simulink model "boat_model_and_controller_inertial"  (R2021a)
settings: Solver=VariableStepAuto  StartTime=0.0  StopTime=20  FixedStep=0.01  RelTol=1e-3
undefined symbols (not defined in the file): ap2, ar2, ay2, bp2, br2, by2, DiscIntNeverNeededParam, Eff, FF_L, FF_R, initial_P, initial_Q, initial_R, initial_uspeed, initial_vspeed, initial_wspeed, initial_Z, Kih, Kir, rear_alfas, T
libraries: simulink x10, dsparch4 x3, pid_lib x1
(part 1 of 2)
settings Model: Creator=Basile  LastModifiedBy=Simão Amaro
settings SolverCC: ConcurrentTasks=on  ZeroCrossAlgorithm=Adaptive  AlgebraicLoopSolver=TrustRegion  PositivePriorityOrder=on
settings DataIOCC: ExternalInput=getinputstruct(op_trim1)  InitialState=getstatestruct(op_trim1)  SaveOutput=off  DSMLogging=off  SaveTime=off  ReturnWorkspaceOutputs=off
settings OptimizationCC: BlockReduction=off  DefaultParameterBehavior=Inlined  UseDivisionForNetSlopeComputation=on  UseFloatMulNetSlope=on  OptimizeBlockIOStorage=off  BufferReuse=off  PassReuseOutputArgsThreshold=0  EfficientFloat2IntCast=on  OptimizeBlockOrder=speed  DifferentSizesBufferReuse=on
settings DebuggingCC: InheritedTsInSrcMsg=none  ParameterTunabilityLossMsg=error  UnconnectedInputMsg=none  UnconnectedOutputMsg=none  UnconnectedLineMsg=none  UniqueDataStoreMsg=error  SFMachineParentedDataDiag=warning  ArithmeticOperatorsInVariantConditions=warning
settings HardwareCC: ProdBitPerLong=64  ProdLongLongMode=on  ProdHWDeviceType=Intel->x86-64 (Linux 64)
settings SFSimCC: SimUseLocalCustomCode=off  MATLABDynamicMemAlloc=off  CustomCodeUndefinedFunction=UseInterfaceOnly
settings RTWCC: Description=Simulink Real-Time  SystemTargetFile=slrealtime.tlc  TemplateMakefile=slrealtime_default_tmf  GenerateReport=on  RTWUseLocalCustomCode=off  Toolchain=Simulink Real-Time Toolchain  BuildConfiguration=Faster Runs  LaunchReport=on  CodeExecutionProfiling=on  TargetLang=C++
settings CodeAppCC: ForceParamTrailComments=on  OperatorAnnotations=on

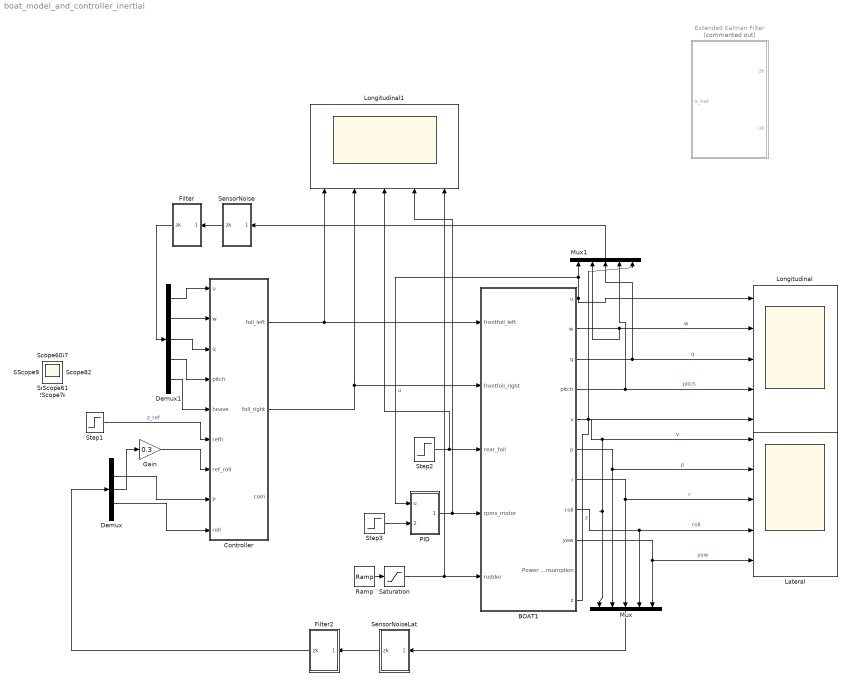
== system boat_model_and_controller_inertial ==
  BOAT1 : Subsystem
  Controller : Subsystem
  Demux : Demux  Outputs=5
  Demux1 : Demux  Outputs=5
  Extended Kalman Filter : Subsystem  Commented=on
  Filter : Subsystem
  Filter2 : Subsystem
  Gain : Gain  Gain=0.3
  Lateral : Scope  NumInputPorts=5
  Longitudinal : Scope  NumInputPorts=5
  Longitudinal1 : Scope  NumInputPorts=5
  Mux : Mux  Inputs=5
  Mux1 : Mux  Inputs=5
  PID : Subsystem
  Ramp : simulink/Sources/Ramp  slope=0  start=0  InitialOutput=15
  Saturation : Saturate  UpperLimit=15  LowerLimit=-15
  SensorNoise : Subsystem
  SensorNoiseLat : Subsystem
  Step1 : Step  Time=0  Before=initial_Z  After=-0.4  SampleTime=0
  Step2 : Step  Time=0  Before=rear_alfas  After=rear_alfas  SampleTime=0
  Step3 : Step  Time=0  Before=initial_uspeed  After=7  SampleTime=0
  Scope{,1..64} (65 alike) : Scope
  wires:
  BOAT1/2(w) -> Mux1/2, Longitudinal/2  "w"
  BOAT1/3(q) -> Mux1/3, Longitudinal/3  "q"
  BOAT1/5(v) -> Mux/1, Lateral/1  "v"
  BOAT1/6(p) -> Lateral/2, Mux/2  "p"
  BOAT1/8(roll) -> Lateral/4, Mux/4  "roll"
  BOAT1/11(z) -> Mux1/5, Longitudinal/5  "z"
  BOAT1/1(u) -> Longitudinal/1, PID/1(u), Mux1/1  "u"
  BOAT1/7(r) -> Lateral/3, Mux/3  "r"
  Demux1/2 -> Controller/2(w)
  Demux1/3 -> Controller/3(q)
  Demux1/4 -> Controller/4(pitch)
  Demux1/5 -> Controller/5(heave)
  Demux1/1 -> Controller/1(u)
  BOAT1/9(yaw) -> Mux/5, Lateral/5  "yaw"
  BOAT1/4(pitch) -> Mux1/4, Longitudinal/4  "pitch"
  Mux1/1 -> SensorNoise/1(states)
  Step1/1 -> Controller/6(refh)  "z_ref"
  Mux/1 -> SensorNoiseLat/1(states)
  Step3/1 -> PID/2(In2)
  Controller/1(foil_left) -> Longitudinal1/1, BOAT1/1(frontfoil_left)
  Controller/2(foil_right) -> Longitudinal1/2, BOAT1/2(frontfoil_right)
  Step2/1 -> Longitudinal1/3, BOAT1/3(rear_foil)
  PID/1(rpms_motor) -> BOAT1/4(rpms_motor), Longitudinal1/4
  Demux/4 -> Controller/9(roll)
  SensorNoise/1(zk) -> Filter/1(states)
  SensorNoiseLat/1(zk) -> Filter2/1(states)
  Filter/1(zk) -> Demux1/1
  Filter2/1(zk) -> Demux/1
  Gain/1 -> Controller/7(ref_roll)
  Demux/2 -> Controller/8(P)
  Demux/3 -> Gain/1
  Ramp/1 -> Saturation/1
  Saturation/1 -> BOAT1/5(rudder), Longitudinal1/5

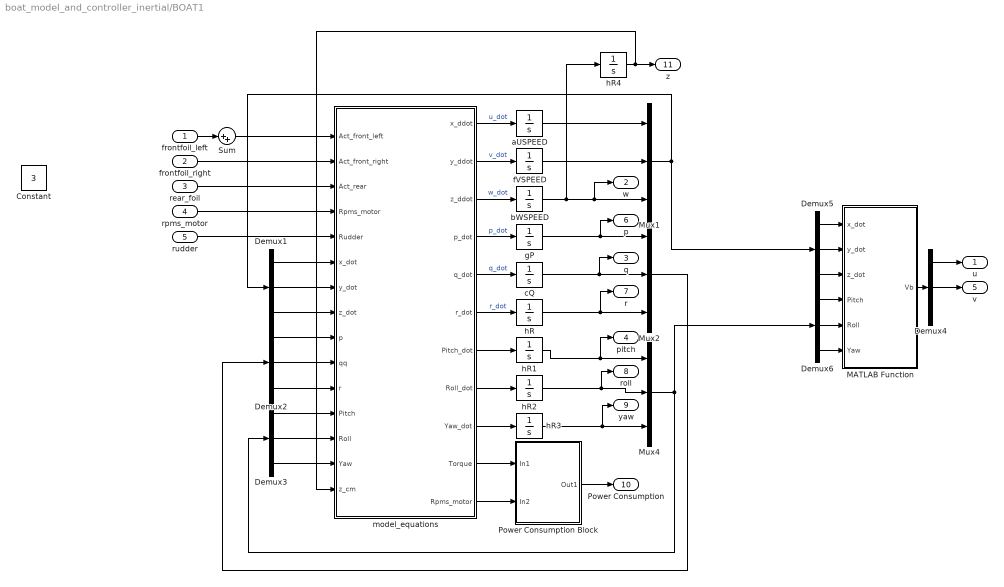
== system boat_model_and_controller_inertial/BOAT1 ==
  frontfoil_left : Inport
  frontfoil_right : Inport  Port=2
  rear_foil : Inport  Port=3
  rpms_motor : Inport  Port=4
  rudder : Inport  Port=5
  Constant : Constant  Value=3
  Demux{1..6} (6 alike) : Demux  Outputs=3
  MATLAB Function : MATLAB Function  TreatAsAtomicUnit=on
  Mux1 : Mux  Inputs=3
  Mux2 : Mux  Inputs=3
  Mux4 : Mux  Inputs=3
  Power Consumption Block : Subsystem
  Sum : Sum  Inputs=|++
  aUSPEED : Integrator  InitialCondition=initial_uspeed
  bWSPEED : Integrator  InitialCondition=initial_wspeed
  cQ : Integrator  InitialCondition=initial_Q
  fVSPEED : Integrator  InitialCondition=initial_vspeed
  gP : Integrator  InitialCondition=initial_P
  hR : Integrator  InitialCondition=initial_R
  hR1 : Integrator
  hR2 : Integrator
  hR3 : Integrator
  hR4 : Integrator  InitialCondition=initial_Z
  model_equations : MATLAB Function  TreatAsAtomicUnit=on  VariantControl=Variant1
  u : Outport  VectorParamsAs1DForOutWhenUnconnected=off
  w : Outport  Port=2  VectorParamsAs1DForOutWhenUnconnected=off
  q : Outport  Port=3  VectorParamsAs1DForOutWhenUnconnected=off
  pitch : Outport  Port=4  VectorParamsAs1DForOutWhenUnconnected=off
  v : Outport  Port=5  VectorParamsAs1DForOutWhenUnconnected=off
  p : Outport  Port=6  VectorParamsAs1DForOutWhenUnconnected=off
  r : Outport  Port=7  VectorParamsAs1DForOutWhenUnconnected=off
  roll : Outport  Port=8  VectorParamsAs1DForOutWhenUnconnected=off
  yaw : Outport  Port=9  VectorParamsAs1DForOutWhenUnconnected=off
  Power Consumption : Outport  Port=10  VectorParamsAs1DForOutWhenUnconnected=off
  z : Outport  Port=11  VectorParamsAs1DForOutWhenUnconnected=off
  wires:
  model_equations/6(r_dot) -> hR/1  "r_dot"
  Mux1/1 -> Demux5/1, Demux1/1
  model_equations/5(q_dot) -> cQ/1  "q_dot"
  rear_foil/1 -> model_equations/3(Act_rear)
  Demux3/2 -> model_equations/13(Roll)
  Demux2/2 -> model_equations/10(qq)
  Demux2/3 -> model_equations/11(r)
  model_equations/4(p_dot) -> gP/1  "p_dot"
  Demux2/1 -> model_equations/9(p)
  rpms_motor/1 -> model_equations/4("Rpms_motor ")
  Demux3/1 -> model_equations/12(Pitch)
  model_equations/2(y_ddot) -> fVSPEED/1  "v_dot"
  Demux1/2 -> model_equations/7(y_dot)
  Mux2/1 -> Demux2/1
  Demux3/3 -> model_equations/14(Yaw)
  model_equations/11(Rpms_motor) -> Power Consumption Block/2(In2)
  Power Consumption Block/1(Out1) -> Power Consumption/1
  model_equations/10(Torque) -> Power Consumption Block/1(In1)
  Demux1/1 -> model_equations/6(x_dot)
  cQ/1 -> q/1, Mux2/2
  hR/1 -> Mux2/3, r/1
  model_equations/3(z_ddot) -> bWSPEED/1  "w_dot"
  model_equations/1(x_ddot) -> aUSPEED/1  "u_dot"
  gP/1 -> p/1, Mux2/1
  model_equations/7(Pitch_dot) -> hR1/1
  model_equations/8(Roll_dot) -> hR2/1
  model_equations/9(Yaw_dot) -> hR3/1
  hR1/1 -> pitch/1, Mux4/1
  hR2/1 -> roll/1, Mux4/2
  hR3/1 -> yaw/1, Mux4/3
  Mux4/1 -> Demux6/1, Demux3/1
  rudder/1 -> model_equations/5(Rudder)
  frontfoil_right/1 -> model_equations/2(Act_front_right)
  frontfoil_left/1 -> Sum/1
  Sum/1 -> model_equations/1(Act_front_left)
  Demux1/3 -> model_equations/8(z_dot)
  fVSPEED/1 -> Mux1/2
  aUSPEED/1 -> Mux1/1
  hR4/1 -> model_equations/15(z_cm), z/1
  bWSPEED/1 -> hR4/1, w/1, Mux1/3
  MATLAB Function/1(Vb) -> Demux4/1
  Demux4/1 -> u/1
  Demux4/2 -> v/1
  Demux5/1 -> MATLAB Function/1(x_dot)
  Demux5/2 -> MATLAB Function/2(y_dot)
  Demux5/3 -> MATLAB Function/3(z_dot)
  Demux6/1 -> MATLAB Function/4(Pitch)
  Demux6/2 -> MATLAB Function/5(Roll)
  Demux6/3 -> MATLAB Function/6(Yaw)

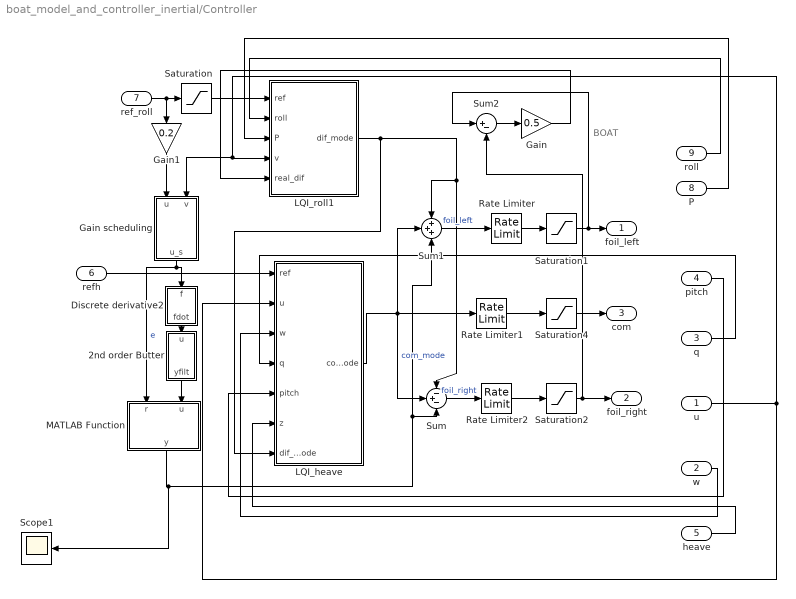
== system boat_model_and_controller_inertial/Controller ==
  note: BOAT
  u : Inport
  w : Inport  Port=2
  q : Inport  Port=3
  pitch : Inport  Port=4
  heave : Inport  Port=5
  refh : Inport  Port=6
  ref_roll : Inport  Port=7
  P : Inport  Port=8
  roll : Inport  Port=9
  2nd order Butter : Subsystem
  Discrete derivative2 : Subsystem
  Gain : Gain  Gain=0.5
  Gain scheduling : MATLAB Function  TreatAsAtomicUnit=on
  Gain1 : Gain  Gain=0.2
  LQI_heave : Subsystem  TreatAsAtomicUnit=on  SystemSampleTime=0.02
      settings: MinAlgLoopOccurrences=on
  LQI_roll1 : Subsystem  TreatAsAtomicUnit=on  SystemSampleTime=0.02
  MATLAB Function : MATLAB Function  TreatAsAtomicUnit=on
  Rate Limiter : RateLimiter  RisingSlewLimit=10  FallingSlewLimit=-10  SampleTimeMode=inherited  InitialCondition=FF_L
  Rate Limiter1 : RateLimiter  RisingSlewLimit=10  FallingSlewLimit=-10  SampleTimeMode=inherited  InitialCondition=FF_L
  Rate Limiter2 : RateLimiter  RisingSlewLimit=10  FallingSlewLimit=-10  SampleTimeMode=inherited  InitialCondition=FF_L
  Saturation : Saturate  UpperLimit=3  LowerLimit=-3
  Saturation1 : Saturate  UpperLimit=14  LowerLimit=-3
  Saturation2 : Saturate  UpperLimit=14  LowerLimit=-3
  Saturation4 : Saturate  UpperLimit=14  LowerLimit=-3
  Scope1 : Scope
  Sum : Sum  Inputs=-+-
  Sum1 : Sum  Inputs=+++
  Sum2 : Sum  Inputs=|+-
  foil_left : Outport  VectorParamsAs1DForOutWhenUnconnected=off
  foil_right : Outport  Port=2  VectorParamsAs1DForOutWhenUnconnected=off
  com : Outport  Port=3  VectorParamsAs1DForOutWhenUnconnected=off
  wires:
  LQI_heave/1(com_mode) -> Rate Limiter1/1, Sum/2, Sum1/2  "com_mode"
  roll/1 -> LQI_roll1/2(roll)
  pitch/1 -> LQI_heave/5(pitch)
  u/1 -> Gain scheduling/2(v), LQI_roll1/4(v), LQI_heave/2(u)
  w/1 -> LQI_heave/3(w)
  P/1 -> LQI_roll1/3(P)
  heave/1 -> LQI_heave/6(z)
  refh/1 -> LQI_heave/1(ref)
  Saturation1/1 -> foil_left/1, Sum2/1
  Saturation4/1 -> com/1
  ref_roll/1 -> Gain1/1, Saturation/1
  LQI_roll1/1(dif_mode) -> LQI_heave/7(dif_mode), Sum/1, Sum1/1
  q/1 -> LQI_heave/4(q)
  Rate Limiter1/1 -> Saturation4/1
  Sum/1 -> Rate Limiter2/1  "foil_right"
  Rate Limiter2/1 -> Saturation2/1
  Gain/1 -> LQI_roll1/5(real_dif)
  Sum2/1 -> Gain/1
  Sum1/1 -> Rate Limiter/1  "foil_left"
  Rate Limiter/1 -> Saturation1/1
  Saturation2/1 -> foil_right/1, Sum2/2
  Gain scheduling/1(u_s) -> Discrete derivative2/1(f), MATLAB Function/1(r)  "e"
  Discrete derivative2/1(fdot) -> 2nd order Butter/1(u)
  Gain1/1 -> Gain scheduling/1(u)
  Saturation/1 -> LQI_roll1/1(ref)
  2nd order Butter/1(yfilt) -> MATLAB Function/2(u)
  MATLAB Function/1(y) -> Scope1/1, Sum/3, Sum1/3

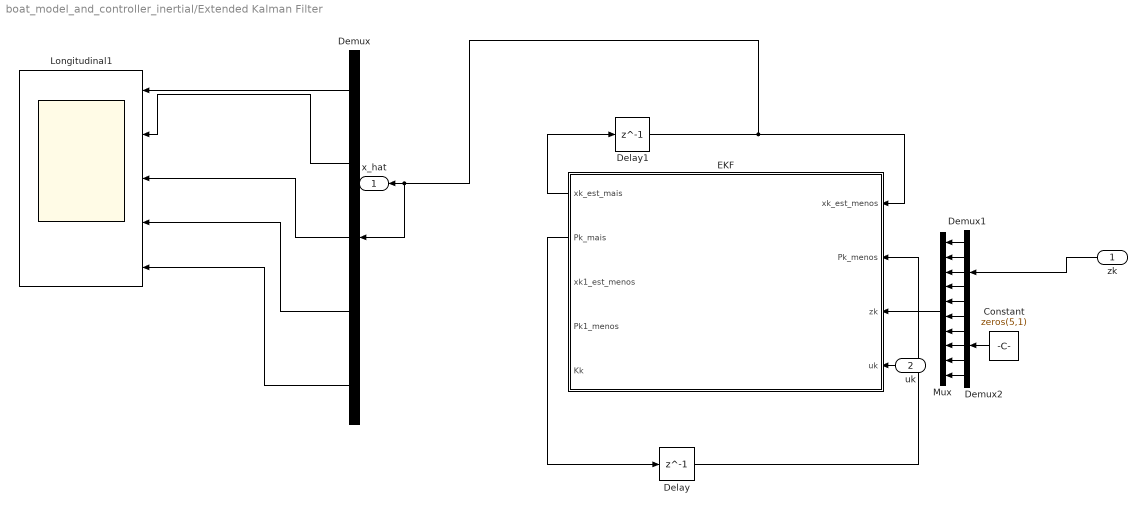
== system boat_model_and_controller_inertial/Extended Kalman Filter ==
  zk : Inport  PortDimensions=5
  uk : Inport  Port=2  PortDimensions=5
  Constant : Constant  Value=zeros(5,1)
  Delay : Delay  DelayLength=1  InitialCondition=1000*eye(37)  SampleTime=0.02
  Delay1 : Delay  DelayLength=1  InitialCondition=[initial_uspeed;0;0;0;initial_Z;0;0;0;0;0;zeros(27,1)]  SampleTime=0.02
  Demux : Demux  Outputs=5
  Demux1 : Demux  Outputs=5
  Demux2 : Demux  Outputs=5
  EKF : MATLAB Function  TreatAsAtomicUnit=on
  Longitudinal1 : Scope  NumInputPorts=5
  Mux : Mux  Inputs=10
  x_hat : Outport
  wires:
  uk/1 -> EKF/4(uk)
  Delay/1 -> EKF/2(Pk_menos)
  Demux/1 -> Longitudinal1/1
  Demux/2 -> Longitudinal1/2
  Demux/3 -> Longitudinal1/3
  Demux/4 -> Longitudinal1/4
  Demux/5 -> Longitudinal1/5
  Delay1/1 -> Demux/1, x_hat/1, EKF/1(xk_est_menos)
  EKF/2(Pk_mais) -> Delay/1
  EKF/1(xk_est_mais) -> Delay1/1
  zk/1 -> Demux1/1
  Mux/1 -> EKF/3(zk)
  Demux1/1 -> Mux/1
  Demux1/2 -> Mux/2
  Demux1/3 -> Mux/3
  Demux1/4 -> Mux/4
  Demux1/5 -> Mux/5
  Demux2/1 -> Mux/6
  Demux2/2 -> Mux/7
  Demux2/3 -> Mux/8
  Demux2/4 -> Mux/9
  Demux2/5 -> Mux/10
  Constant/1 -> Demux2/1

== system boat_model_and_controller_inertial/Filter ==
  states : Inport
  2nd order Butter : Subsystem
  Demux2 : Demux  Outputs=5
  Longitudinal1 : Scope  NumInputPorts=5
  Mux1 : Mux  Inputs=2
  Mux2 : Mux  Inputs=5
  zk : Outport
  wires:
  states/1 -> Demux2/1
  Mux2/1 -> zk/1
  Demux2/1 -> Mux2/1
  Demux2/2 -> Mux2/2
  Demux2/4 -> Mux2/4
  Demux2/5 -> Mux2/5
  Mux1/1 -> Longitudinal1/3
  2nd order Butter/1(yfilt) -> Mux1/1, Mux2/3
  Demux2/3 -> Mux1/2, 2nd order Butter/1(u)  "q"

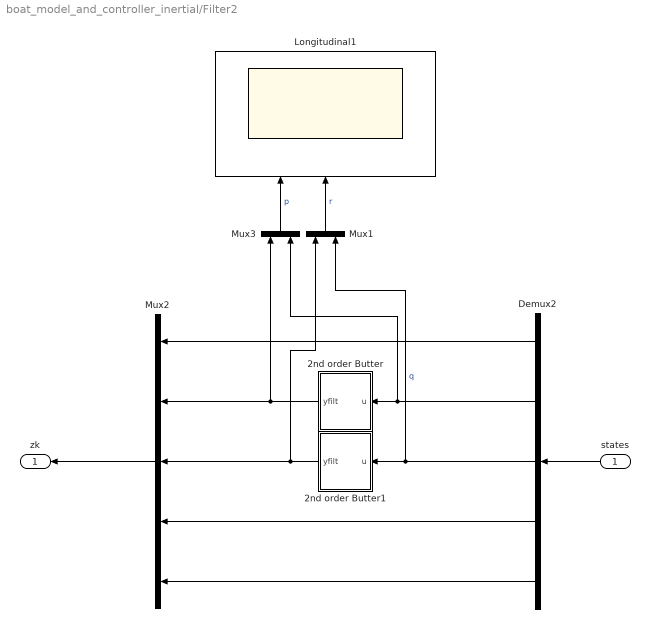
== system boat_model_and_controller_inertial/Filter2 ==
  states : Inport
  2nd order Butter : Subsystem
  2nd order Butter1 : Subsystem
  Demux2 : Demux  Outputs=5
  Longitudinal1 : Scope  NumInputPorts=5
  Mux1 : Mux  Inputs=2
  Mux2 : Mux  Inputs=5
  Mux3 : Mux  Inputs=2
  zk : Outport
  wires:
  states/1 -> Demux2/1
  Mux2/1 -> zk/1
  Demux2/1 -> Mux2/1
  Demux2/4 -> Mux2/4
  Demux2/5 -> Mux2/5
  Demux2/2 -> Mux3/2, 2nd order Butter/1(u)
  2nd order Butter/1(yfilt) -> Mux3/1, Mux2/2
  2nd order Butter1/1(yfilt) -> Mux1/1, Mux2/3
  Demux2/3 -> Mux1/2, 2nd order Butter1/1(u)  "q"
  Mux1/1 -> Longitudinal1/3  "r"
  Mux3/1 -> Longitudinal1/2  "p"

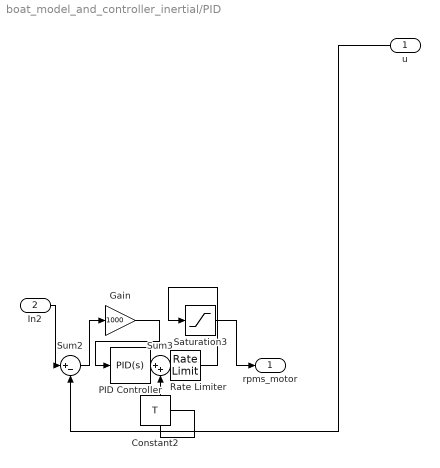
== system boat_model_and_controller_inertial/PID ==
  u : Inport
  In2 : Inport  Port=2
  Constant2 : Constant  Value=T
  Gain : Gain  Gain=1000
  PID Controller : pid_lib/PID Controller  Controller=PID  Form=Parallel  TimeDomain=Continuous-time  UseExternalTs=off  SampleTime=-1  IntegratorMethod=Forward Euler  FilterMethod=Forward Euler  ControllerParametersSource=internal  P=1  I=1  D=0.00001  UseFilter=on  N=100  TunerSelectOption=Transfer Function Based (PID Tuner App)  InitialConditionSource=internal  InitialConditionForIntegrator=0  InitialConditionForFilter=0  DifferentiatorICPrevScaledInput=0  ExternalReset=none  TrackingMode=off  Kt=1  LimitOutput=off  SatLimitsSource=internal  UpperSaturationLimit=inf  LowerSaturationLimit=-inf  LinearizeAsGain=on  AntiWindupMode=none  Kb=1  POutMin=[]  POutMax=[]  IOutMin=[]  IOutMax=[]  DOutMin=[]  DOutMax=[]  NOutMin=[]  NOutMax=[]  SumOutMin=[]  SumOutMax=[]  SaturationOutMin=[]  SaturationOutMax=[]  PParamMin=[]  PParamMax=[]  IParamMin=[]  IParamMax=[]  DParamMin=[]  DParamMax=[]  NParamMin=[]  NParamMax=[]  KbParamMin=[]  KbParamMax=[]  KtParamMin=[]  KtParamMax=[]  KbOutMin=[]  KbOutMax=[]  KtOutMin=[]  KtOutMax=[]  IntegratorOutMin=[]  IntegratorOutMax=[]  FilterOutMin=[]  FilterOutMax=[]  SumI1OutMin=[]  SumI1OutMax=[]  SumI2OutMin=[]  SumI2OutMax=[]  SumI3OutMin=[]  SumI3OutMax=[]  SumI4OutMin=[]  SumI4OutMax=[]  SumDOutMin=[]  SumDOutMax=[]  DifferentiatorOutMin=[]  DifferentiatorOutMax=[]  FilterDiffOutCoefMin=[]  FilterDiffOutCoefMax=[]  ReciprocalOutMin=[]  ReciprocalOutMax=[]  SumDenOutMin=[]  SumDenOutMax=[]  SumNumOutMin=[]  SumNumOutMax=[]  DivideOutMin=[]  DivideOutMax=[]  UdiffTsProdOutMin=[]  UdiffTsProdOutMax=[]  NTsProdOutMin=[]  NTsProdOutMax=[]  UintegralTsProdOutMin=[]  UintegralTsProdOutMax=[]  UngainTsProdOutMin=[]  UngainTsProdOutMax=[]  IntegratorContinuousStateAttributes=''  IntegratorStateMustResolveToSignalObject=off  IntegratorRTWStateStorageClass=Auto  FilterContinuousStateAttributes=''  FilterStateMustResolveToSignalObject=off  FilterRTWStateStorageClass=Auto  ParallelPVariant=InternalParameters  IdealPVariant=Disabled  IVariant=InternalParameters  DVariant=InternalParameters  IntegratorVariant=Continuous  SatVariant=Disabled  AWVariant=Passthrough  PCopyVariant=Disabled  TRVariant=Disabled  FdbkBlocksVariant=Forward  IdealPFdbkVariant=Disabled  SatFdbkVariant=Disabled  DerivativeFilterVariant=ContFilter  NVariant=InternalParameters  NCopyVariant=Disabled  FilterICVariant=InternalICsFilter  IntegratorICVariant=InternalICs  ExternalResetVariant=Disabled  TRSumVariant=Passthrough  SumFdbkVariant=Disabled  SumVariant=Sum_PID  TsampFilterVariant=InternalTs  TsampNgainVariant=Passthrough  TsampIntegralVariant=Passthrough  ExternalSaturationOutDataTypeStr=Inherit: Same as second input
  Rate Limiter : RateLimiter  RisingSlewLimit=1000  FallingSlewLimit=-1000  SampleTimeMode=inherited  InitialCondition=T
  Saturation3 : Saturate  UpperLimit=9000
  Sum2 : Sum  Inputs=|+-
  Sum3 : Sum  Inputs=|++
  rpms_motor : Outport
  wires:
  u/1 -> Sum2/2
  Sum3/1 -> Rate Limiter/1
  Gain/1 -> PID Controller/1
  Saturation3/1 -> rpms_motor/1
  PID Controller/1 -> Sum3/1
  Rate Limiter/1 -> Saturation3/1
  Sum2/1 -> Gain/1
  In2/1 -> Sum2/1
  Constant2/1 -> Sum3/2

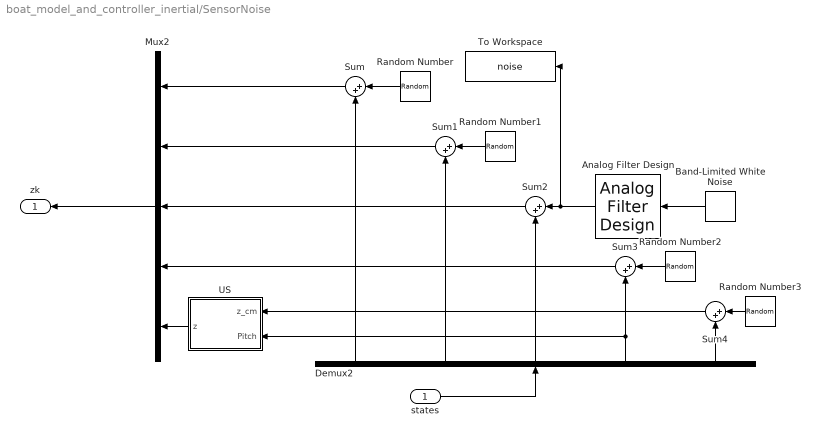
== system boat_model_and_controller_inertial/SensorNoise ==
  states : Inport
  Analog Filter Design : dsparch4/Analog Filter Design  method=Butterworth  filttype=Highpass  N=8  Wlo=3*2*pi  Whi=80  Rp=2  Rs=40
  Band-Limited White Noise : simulink/Sources/Band-Limited White Noise  Cov=[0.05]  Ts=0.02  seed=[23341]
  Demux2 : Demux  Outputs=5
  Mux2 : Mux  Inputs=5
  Random Number : RandomNumber  Variance=0.001^2  Seed=31233  SampleTime=0.02
  Random Number1 : RandomNumber  Variance=0.001^2  Seed=31232  SampleTime=0.02
  Random Number2 : RandomNumber  Variance=0.005^2  Seed=372323  SampleTime=0.02
  Random Number3 : RandomNumber  Variance=0.0005^2  Seed=312392  SampleTime=0.02
  Sum{,1..4} (5 alike) : Sum  Inputs=|++
  To Workspace : ToWorkspace  VariableName=noise  SaveFormat=Timeseries  SampleTime=0.02
  US : MATLAB Function  TreatAsAtomicUnit=on
  zk : Outport
  wires:
  Demux2/1 -> Sum/2
  Random Number2/1 -> Sum3/1
  Random Number3/1 -> Sum4/1
  Random Number/1 -> Sum/1
  Demux2/4 -> Sum3/2, US/2(Pitch)
  Demux2/3 -> Sum2/2
  Demux2/5 -> Sum4/2
  Demux2/2 -> Sum1/2
  Random Number1/1 -> Sum1/1
  states/1 -> Demux2/1
  Mux2/1 -> zk/1
  Sum/1 -> Mux2/1
  Sum1/1 -> Mux2/2
  Sum2/1 -> Mux2/3
  Sum3/1 -> Mux2/4
  US/1(z) -> Mux2/5
  Sum4/1 -> US/1(z_cm)
  Analog Filter Design/1 -> To Workspace/1, Sum2/1
  Band-Limited White Noise/1 -> Analog Filter Design/1

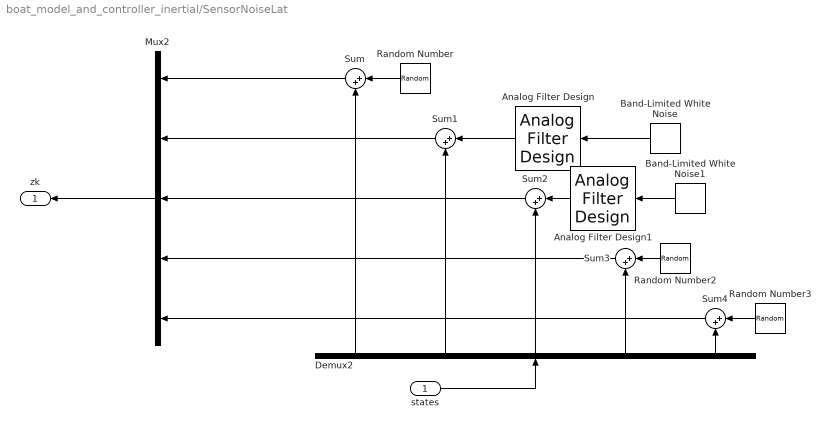
== system boat_model_and_controller_inertial/SensorNoiseLat ==
  states : Inport
  Analog Filter Design : dsparch4/Analog Filter Design  method=Butterworth  filttype=Highpass  N=8  Wlo=15*2*pi  Whi=80  Rp=2  Rs=40
  Analog Filter Design1 : dsparch4/Analog Filter Design  method=Butterworth  filttype=Highpass  N=8  Wlo=3*2*pi  Whi=80  Rp=2  Rs=40
  Band-Limited White Noise : simulink/Sources/Band-Limited White Noise  Cov=[0.0000000001]  Ts=0.02  seed=[23341]
  Band-Limited White Noise1 : simulink/Sources/Band-Limited White Noise  Cov=[0.00005]  Ts=0.02  seed=[23341]
  Demux2 : Demux  Outputs=5
  Mux2 : Mux  Inputs=5
  Random Number : RandomNumber  Variance=0.05^2  Seed=31233  SampleTime=0.02
  Random Number2 : RandomNumber  Variance=0.005^2  Seed=372323  SampleTime=0.02
  Random Number3 : RandomNumber  Variance=0.005^2  Seed=312392  SampleTime=0.02
  Sum{,1..4} (5 alike) : Sum  Inputs=|++
  zk : Outport
  wires:
  Demux2/1 -> Sum/2
  Random Number2/1 -> Sum3/1
  Random Number3/1 -> Sum4/1
  Random Number/1 -> Sum/1
  Demux2/4 -> Sum3/2
  Demux2/3 -> Sum2/2
  Demux2/5 -> Sum4/2
  Demux2/2 -> Sum1/2
  states/1 -> Demux2/1
  Mux2/1 -> zk/1
  Sum/1 -> Mux2/1
  Sum1/1 -> Mux2/2
  Sum2/1 -> Mux2/3
  Sum3/1 -> Mux2/4
  Sum4/1 -> Mux2/5
  Band-Limited White Noise/1 -> Analog Filter Design/1
  Band-Limited White Noise1/1 -> Analog Filter Design1/1
  Analog Filter Design1/1 -> Sum2/1
  Analog Filter Design/1 -> Sum1/1

== system boat_model_and_controller_inertial/BOAT1/Power Consumption Block ==
  In1 : Inport
  In2 : Inport  Port=2
  2-D Lookup Table : Lookup_n-D  BreakpointsForDimension1=[1:6000]  BreakpointsForDimension2=[1:140]  Table=Eff  InternalRulePriority=Speed  RndMeth=Simplest  InputSameDT=on
      settings: InputPortMap=u0,u1
  Gain : Gain  Gain=10
  MATLAB Function1 : MATLAB Function  TreatAsAtomicUnit=on
  Out1 : Outport
  wires:
  In2/1 -> 2-D Lookup Table/1, MATLAB Function1/2(Rpms_motor)
  MATLAB Function1/1(P_elec) -> Out1/1
  In1/1 -> Gain/1, MATLAB Function1/1(Torque)
  Gain/1 -> 2-D Lookup Table/2
  2-D Lookup Table/1 -> MATLAB Function1/3(Eficiencia_motor)

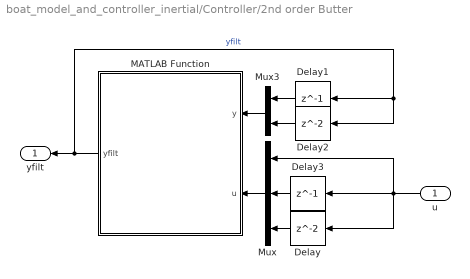
== system boat_model_and_controller_inertial/Controller/2nd order Butter ==
  u : Inport
  Delay : Delay
  Delay1 : Delay  DelayLength=1  SampleTime=0.02
  Delay2 : Delay
  Delay3 : Delay  DelayLength=1  SampleTime=0.02
  MATLAB Function : MATLAB Function  TreatAsAtomicUnit=on
  Mux : Mux  Inputs=3
  Mux3 : Mux  Inputs=2
  yfilt : Outport
  wires:
  Mux3/1 -> MATLAB Function/1(y)
  Mux/1 -> MATLAB Function/2(u)
  MATLAB Function/1(yfilt) -> Delay1/1, Delay2/1, yfilt/1  "yfilt"
  Delay/1 -> Mux/3
  Delay3/1 -> Mux/2
  u/1 -> Mux/1, Delay3/1, Delay/1
  Delay1/1 -> Mux3/1
  Delay2/1 -> Mux3/2

== system boat_model_and_controller_inertial/Controller/Discrete derivative2 ==
  f : Inport
  Constant : Constant  Value=0
  Discrete Derivative : simulink/Discrete/Discrete Derivative  gainval=1.0  ICPrevScaledInput=0.0  OutMin=[]  OutMax=[]  OutDataType=fixdt(1, 16)  OutScaling=2^-10  DoSatur=off
  Step : Step  Time=0.01  Before=-1
  Switch : Switch  Criteria=u2 > Threshold
  fdot : Outport  VectorParamsAs1DForOutWhenUnconnected=off
  wires:
  Discrete Derivative/1 -> Switch/1  "ddtkz"
  Constant/1 -> Switch/3
  Step/1 -> Switch/2
  f/1 -> Discrete Derivative/1
  Switch/1 -> fdot/1

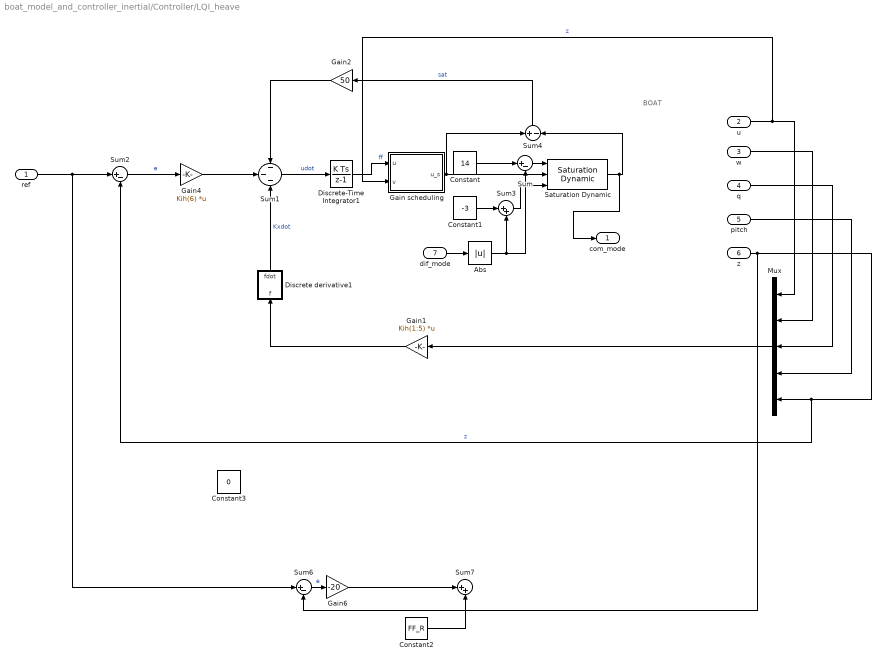
== system boat_model_and_controller_inertial/Controller/LQI_heave ==
  note: BOAT
  ref : Inport
  u : Inport  Port=2
  w : Inport  Port=3
  q : Inport  Port=4
  pitch : Inport  Port=5
  z : Inport  Port=6
  dif_mode : Inport  Port=7
  Abs : Abs
  Constant : Constant  Value=14
  Constant1 : Constant  Value=-3
  Constant2 : Constant  Value=FF_R
  Constant3 : Constant  Value=0
  Discrete derivative1 : Subsystem
  Discrete-Time Integrator1 : DiscreteIntegrator  gainval=1  InitialCondition=FF_R  SampleTime=-1  ICPrevOutput=DiscIntNeverNeededParam  ICPrevScaledInput=DiscIntNeverNeededParam
  Gain scheduling : MATLAB Function  TreatAsAtomicUnit=on
  Gain1 : Gain  Gain=Kih(1:5)  Multiplication=Matrix(K*u)
  Gain2 : Gain  Gain=50
  Gain4 : Gain  Gain=Kih(6)  Multiplication=Matrix(K*u)
  Gain6 : Gain  Gain=-20
  Mux : Mux  Inputs=5
  Saturation Dynamic : simulink/Discontinuities/Saturation Dynamic  OutMin=[]  OutMax=[]  OutDataTypeStr=Inherit: Same as second input  OutDataType=fixdt(1, 16)  OutScaling=2^-10  DoSatur=off
  Sum : Sum  Inputs=|+-
  Sum1 : Sum  Inputs=---
  Sum2 : Sum  Inputs=|+-
  Sum3 : Sum  Inputs=|++
  Sum4 : Sum  Inputs=+|-
  Sum6 : Sum  Inputs=|+-
  Sum7 : Sum  Inputs=|++
  com_mode : Outport  VectorParamsAs1DForOutWhenUnconnected=off
  wires:
  Sum4/1 -> Gain2/1  "sat"
  Gain2/1 -> Sum1/1
  Sum1/1 -> Discrete-Time Integrator1/1  "udot"
  w/1 -> Mux/2
  q/1 -> Mux/3
  pitch/1 -> Mux/4
  u/1 -> Gain scheduling/2(v), Mux/1  "z"
  z/1 -> Mux/5, Sum2/2, Sum6/2  "z"
  Gain1/1 -> Discrete derivative1/1(f)
  Mux/1 -> Gain1/1
  Discrete derivative1/1(fdot) -> Sum1/3  "Kxdot"
  Gain4/1 -> Sum1/2
  Sum2/1 -> Gain4/1  "e"
  Discrete-Time Integrator1/1 -> Gain scheduling/1(u)  "ff"
  Gain scheduling/1(u_s) -> Saturation Dynamic/2, Sum4/1
  Sum/1 -> Saturation Dynamic/1
  Constant/1 -> Sum/1
  dif_mode/1 -> Abs/1
  Abs/1 -> Sum/2, Sum3/2
  Sum3/1 -> Saturation Dynamic/3
  Constant1/1 -> Sum3/1
  ref/1 -> Sum6/1, Sum2/1
  Constant2/1 -> Sum7/2
  Saturation Dynamic/1 -> com_mode/1, Sum4/2
  Gain6/1 -> Sum7/1
  Sum6/1 -> Gain6/1  "e"

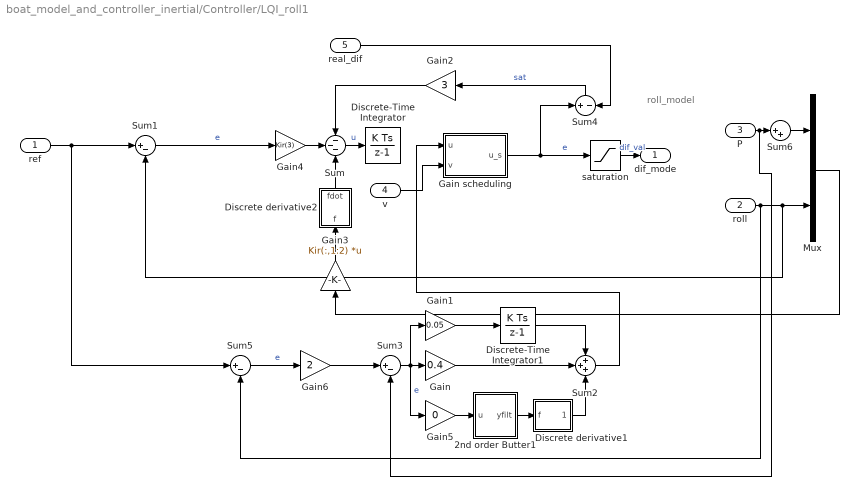
== system boat_model_and_controller_inertial/Controller/LQI_roll1 ==
  note: roll_model
  ref : Inport
  roll : Inport  Port=2
  P : Inport  Port=3
  v : Inport  Port=4
  real_dif : Inport  Port=5
  2nd order Butter1 : Subsystem
  Discrete derivative1 : Subsystem
  Discrete derivative2 : Subsystem
  Discrete-Time Integrator : DiscreteIntegrator  gainval=1  SampleTime=-1  ICPrevOutput=DiscIntNeverNeededParam  ICPrevScaledInput=DiscIntNeverNeededParam
  Discrete-Time Integrator1 : DiscreteIntegrator  gainval=1  SampleTime=0.02  LimitOutput=on  UpperSaturationLimit=5  LowerSaturationLimit=-5  ICPrevOutput=DiscIntNeverNeededParam  ICPrevScaledInput=DiscIntNeverNeededParam
  Gain : Gain  Gain=0.4
  Gain scheduling : MATLAB Function  TreatAsAtomicUnit=on
  Gain1 : Gain  Gain=0.05
  Gain2 : Gain  Gain=3
  Gain3 : Gain  Gain=Kir(:,1:2)  Multiplication=Matrix(K*u)
  Gain4 : Gain  Gain=Kir(3)
  Gain5 : Gain  Gain=0
  Gain6 : Gain  Gain=2
  Mux : Mux  Inputs=2
  Sum : Sum  Inputs=---
  Sum1 : Sum  Inputs=|+-
  Sum2 : Sum  Inputs=+++
  Sum3 : Sum  Inputs=|+-
  Sum4 : Sum  Inputs=+|-
  Sum5 : Sum  Inputs=|+-
  Sum6 : Sum  Inputs=|++
  saturation : Saturate  UpperLimit=8.5  LowerLimit=-8.5
  dif_mode : Outport  VectorParamsAs1DForOutWhenUnconnected=off
  wires:
  Sum1/1 -> Gain4/1  "e"
  Sum4/1 -> Gain2/1  "sat"
  Gain3/1 -> Discrete derivative2/1(f)
  Gain2/1 -> Sum/1
  Mux/1 -> Gain3/1
  Sum/1 -> Discrete-Time Integrator/1  "u"
  Gain4/1 -> Sum/2
  Discrete derivative2/1(fdot) -> Sum/3
  real_dif/1 -> Sum4/2
  Sum3/1 -> Gain5/1, Gain1/1, Gain/1  "e"
  roll/1 -> Sum5/2, Sum1/2, Mux/2
  Sum5/1 -> Gain6/1  "e"
  ref/1 -> Sum5/1, Sum1/1
  saturation/1 -> dif_mode/1  "dif_val"
  P/1 -> Sum3/2, Sum6/1
  Sum6/1 -> Mux/1
  v/1 -> Gain scheduling/2(v)
  Gain6/1 -> Sum3/1
  Discrete-Time Integrator1/1 -> Sum2/1
  Gain/1 -> Sum2/2
  Gain1/1 -> Discrete-Time Integrator1/1
  Gain5/1 -> 2nd order Butter1/1(u)
  2nd order Butter1/1(yfilt) -> Discrete derivative1/1(f)
  Discrete derivative1/1(fdot) -> Sum2/3
  Gain scheduling/1(u_s) -> saturation/1, Sum4/1  "e"
  Sum2/1 -> Gain scheduling/1(u)

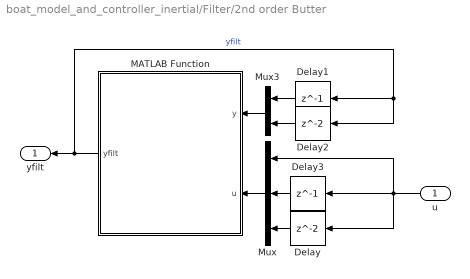
== system boat_model_and_controller_inertial/Filter/2nd order Butter ==
  u : Inport
  Delay : Delay
  Delay1 : Delay  DelayLength=1  SampleTime=0.02
  Delay2 : Delay
  Delay3 : Delay  DelayLength=1  SampleTime=0.02
  MATLAB Function : MATLAB Function  TreatAsAtomicUnit=on
  Mux : Mux  Inputs=3
  Mux3 : Mux  Inputs=2
  yfilt : Outport
  wires:
  Mux3/1 -> MATLAB Function/1(y)
  Mux/1 -> MATLAB Function/2(u)
  MATLAB Function/1(yfilt) -> Delay1/1, Delay2/1, yfilt/1  "yfilt"
  Delay/1 -> Mux/3
  Delay3/1 -> Mux/2
  u/1 -> Mux/1, Delay3/1, Delay/1
  Delay1/1 -> Mux3/1
  Delay2/1 -> Mux3/2

== system boat_model_and_controller_inertial/Filter2/2nd order Butter ==
  u : Inport
  Delay : Delay
  Delay1 : Delay  DelayLength=1  SampleTime=0.02
  Delay2 : Delay
  Delay3 : Delay  DelayLength=1  SampleTime=0.02
  MATLAB Function : MATLAB Function  TreatAsAtomicUnit=on
  Mux : Mux  Inputs=3
  Mux3 : Mux  Inputs=2
  yfilt : Outport
  wires:
  Mux3/1 -> MATLAB Function/1(y)
  Mux/1 -> MATLAB Function/2(u)
  MATLAB Function/1(yfilt) -> Delay1/1, Delay2/1, yfilt/1  "yfilt"
  Delay/1 -> Mux/3
  Delay3/1 -> Mux/2
  u/1 -> Mux/1, Delay3/1, Delay/1
  Delay1/1 -> Mux3/1
  Delay2/1 -> Mux3/2

== system boat_model_and_controller_inertial/Filter2/2nd order Butter1 ==
  u : Inport
  Delay : Delay
  Delay1 : Delay  DelayLength=1  SampleTime=0.02
  Delay2 : Delay
  Delay3 : Delay  DelayLength=1  SampleTime=0.02
  MATLAB Function : MATLAB Function  TreatAsAtomicUnit=on
  Mux : Mux  Inputs=3
  Mux3 : Mux  Inputs=2
  yfilt : Outport
  wires:
  Mux3/1 -> MATLAB Function/1(y)
  Mux/1 -> MATLAB Function/2(u)
  MATLAB Function/1(yfilt) -> Delay1/1, Delay2/1, yfilt/1  "yfilt"
  Delay/1 -> Mux/3
  Delay3/1 -> Mux/2
  u/1 -> Mux/1, Delay3/1, Delay/1
  Delay1/1 -> Mux3/1
  Delay2/1 -> Mux3/2

== system boat_model_and_controller_inertial/Controller/LQI_heave/Discrete derivative1 ==
  f : Inport
  Abs : Abs  Commented=on
  Constant : Constant  Value=0
  Discrete Derivative : simulink/Discrete/Discrete Derivative  gainval=1.0  ICPrevScaledInput=0.0  OutMin=[]  OutMax=[]  OutDataType=fixdt(1, 16)  OutScaling=2^-10  DoSatur=off
  Discrete Derivative1 : simulink/Discrete/Discrete Derivative  Commented=on  gainval=1.0  ICPrevScaledInput=0.0  OutMin=[]  OutMax=[]  OutDataType=fixdt(1, 16)  OutScaling=2^-10  DoSatur=off
  Step : Step  Time=0.01  Before=-1
  Switch : Switch  Criteria=u2 > Threshold
  fdot : Outport  VectorParamsAs1DForOutWhenUnconnected=off
  wires:
  Switch/1 -> fdot/1
  f/1 -> Discrete Derivative/1
  Constant/1 -> Switch/3
  Discrete Derivative/1 -> Switch/1  "ddtkz"
  ? -> Discrete Derivative1/1
  Discrete Derivative1/1 -> Abs/1
  Step/1 -> Switch/2

== system boat_model_and_controller_inertial/Controller/LQI_roll1/2nd order Butter1 ==
  u : Inport
  Delay : Delay
  Delay1 : Delay  DelayLength=1  SampleTime=0.02
  Delay2 : Delay
  Delay3 : Delay  DelayLength=1  SampleTime=0.02
  MATLAB Function : MATLAB Function  TreatAsAtomicUnit=on
  Mux : Mux  Inputs=3
  Mux3 : Mux  Inputs=2
  yfilt : Outport
  wires:
  Mux3/1 -> MATLAB Function/1(y)
  Mux/1 -> MATLAB Function/2(u)
  MATLAB Function/1(yfilt) -> Delay1/1, Delay2/1, yfilt/1  "yfilt"
  Delay/1 -> Mux/3
  Delay3/1 -> Mux/2
  u/1 -> Mux/1, Delay3/1, Delay/1
  Delay1/1 -> Mux3/1
  Delay2/1 -> Mux3/2

== system boat_model_and_controller_inertial/Controller/LQI_roll1/Discrete derivative1 ==
  f : Inport
  Constant : Constant  Value=0
  Discrete Derivative : simulink/Discrete/Discrete Derivative  gainval=1.0  ICPrevScaledInput=0.0  OutMin=[]  OutMax=[]  OutDataType=fixdt(1, 16)  OutScaling=2^-10  DoSatur=off
  Step : Step  Time=0.01  Before=-1
  Switch : Switch  Criteria=u2 > Threshold
  fdot : Outport  VectorParamsAs1DForOutWhenUnconnected=off
  wires:
  Discrete Derivative/1 -> Switch/1  "ddtkz"
  Constant/1 -> Switch/3
  Step/1 -> Switch/2
  f/1 -> Discrete Derivative/1
  Switch/1 -> fdot/1

== system boat_model_and_controller_inertial/Controller/LQI_roll1/Discrete derivative2 ==
  f : Inport
  Constant : Constant  Value=0
  Discrete Derivative : simulink/Discrete/Discrete Derivative  gainval=1.0  ICPrevScaledInput=0.0  OutMin=[]  OutMax=[]  OutDataType=fixdt(1, 16)  OutScaling=2^-10  DoSatur=off
  Step : Step  Time=0.01  Before=-1
  Switch : Switch  Criteria=u2 > Threshold
  fdot : Outport  VectorParamsAs1DForOutWhenUnconnected=off
  wires:
  Discrete Derivative/1 -> Switch/1  "ddtkz"
  Constant/1 -> Switch/3
  Step/1 -> Switch/2
  f/1 -> Discrete Derivative/1
  Switch/1 -> fdot/1

== matlab function boat_model_and_controller_inertial/Controller/LQI_roll1/Gain scheduling ==
  data: u input; u_s output; v input
function u_s = fcn(u,v)
v_ref = 6.4;
if(v>v_ref)
    u_s = u*v_ref^2/v^2;
else
    u_s = u;
end

== matlab function boat_model_and_controller_inertial/SensorNoise/US ==
  data: z_cm input; z output; Pitch input
function z = fcn(z_cm,Pitch)
Roll = 0; %Approximation
dist_cm_Us_x = 3.150;   %distance between cm and US
z = (z_cm*cosd(Roll)-tand(Pitch)*dist_cm_Us_x)/cosd(Pitch);

== matlab function boat_model_and_controller_inertial/Controller/LQI_heave/Gain scheduling ==
  data: u input; u_s output; v input
function u_s = fcn(u,v)
v_ref = 6.4;
if(v>v_ref)
    u_s = u*v_ref^2/v^2;
else
    u_s = u;
end

== matlab function boat_model_and_controller_inertial/Filter/2nd order Butter/MATLAB Function ==
  data: y input; u input; yfilt output; bp2 parameter; ap2 parameter
function yfilt = filtit(y,u, bp2, ap2)
b = bp2;
a = ap2;
yfilt = 0;
for i=1:length(u)
   yfilt = yfilt + b(i)*u(i);
end

for i=2:length(y)+1
   yfilt = yfilt - a(i)*y(i-1); 
end

yfilt = yfilt/a(1);

end

== matlab function boat_model_and_controller_inertial/Controller/LQI_roll1/2nd order Butter1/MATLAB Function ==
  data: y input; u input; yfilt output; by2 parameter; ay2 parameter
function yfilt = filtit(y,u, by2, ay2)
b = by2;
a = ay2;
yfilt = 0;
for i=1:length(u)
   yfilt = yfilt + b(i)*u(i);
end

for i=2:length(y)+1
   yfilt = yfilt - a(i)*y(i-1); 
end

yfilt = yfilt/a(1);

end

== matlab function boat_model_and_controller_inertial/Filter2/2nd order Butter/MATLAB Function ==
  data: y input; u input; yfilt output; br2 parameter; ar2 parameter
function yfilt = filtit(y,u, br2, ar2)
b = br2;
a = ar2;
yfilt = 0;
for i=1:length(u)
   yfilt = yfilt + b(i)*u(i);
end

for i=2:length(y)+1
   yfilt = yfilt - a(i)*y(i-1); 
end

yfilt = yfilt/a(1);

end

== matlab function boat_model_and_controller_inertial/Extended Kalman Filter/EKF ==
  data: xk_est_mais output; xk_est_menos input; Pk_menos input; zk input; Pk_mais output; xk1_est_menos output; Pk1_menos output; Kk output; uk input
function [xk_est_mais,Pk_mais,xk1_est_menos,Pk1_menos,Kk] = extended_kalman_filter(xk_est_menos,Pk_menos,zk,uk)

%EKF matrices
Rk = diag([0.05^2 0.05^2 0.25^2 0.25^2 0.005^2 0 0 0 0 0]); 
Qku = eye(10); %Quando tiver erro de modelo

%% RKM Aproximation

%Prediction Phase
%Phik = Jacobian_func_out(xk_est_menos(1),xk_est_menos(2),xk_est_menos(3),xk_est_menos(4),xk_est_menos(5),xk_est_menos(6),xk_est_menos(7),xk_est_menos(8),xk_est_menos(9),uk(3),uk(2),uk(1),uk(4),uk(5));
Phik = fwjac(xk,uk);
Phik = expm(Phik*0.02);
Qk = Phik*Qku*Phik'*0.02;
xk1_est_menos = RKM_EKF(xk_est_menos,uk);
Pk1_menos = Phik*Pk_menos*Phik'+Qk;

%Correction Phase
yk = xk1_est_menos;
Hk = Hk_func(xk1_est_menos(4),xk1_est_menos(5),xk1_est_menos(9));
yk(5) = (yk(5)*cosd(yk(9))-tand(yk(4))*dist_cm_Us_x)/cosd(yk(4)); 
Kk = Pk1_menos*Hk'*inv(Hk*Pk1_menos*Hk'+Rk);
xk_est_mais = xk1_est_menos+Kk*(zk-yk);
Pk_mais = (eye(10)-Kk*Hk)*Pk1_menos*(eye(10)-Kk*Hk)'+Kk*Rk*Kk';
end

== matlab function boat_model_and_controller_inertial/BOAT1/Power Consumption Block/MATLAB Function1 ==
  data: Torque input; P_elec output; Rpms_motor input; Eficiencia_motor input
function P_elec = fcn(Torque,Rpms_motor,Eficiencia_motor)
P_mec = Torque*Rpms_motor*2*pi/60;
P_elec = P_mec/Eficiencia_motor;
